simulink model "WOTC_simulation"  (R2024b)
settings: Solver=ode4  StartTime=0.0  StopTime=4700  FixedStep=0.01  RelTol=1e-3
InitFcn:
  | % Clear all variables from the workspace to ensure a clean start
  | clearvars;
  | 
  | % Run the setup script to load fresh parameters
  | run('models/osvData.m');
  | 
  | % Print a message to the command window to confirm
  | disp('Workspace cleared and initial variables loaded.');
StopFcn:
  | % Folder name
  | saveFolder = 'output data/';
  | timestamp = string(datetime('now', 'Format', 'yyyyMMdd_HHmmss'));
  | 
  | %make folder for simulation run data
  | mkdir(saveFolder + timestamp);
  | 
  | filePath = saveFolder + timestamp + "/" + timestamp + ".mat";
  | 
  | % 3. SAVE the file to the specified location
  | save(filePath, 'out');
  | 
  | disp(['Simulation data saved to: ' filePath]);
undefined symbols (not defined in the file or in its folder): osvData, vessel
libraries: wopc_lib x23, mssSimulink x6, simulink_extras x3, dspsigops x1, SignalEditorBlockLib x1
settings Model: PauseTimes=0  PacingRate=0.010000  Creator=lenna  LastModifiedBy=lenna
settings ModelReferenceCC: EnableRefExpFcnMdlSchedulingChecks=on

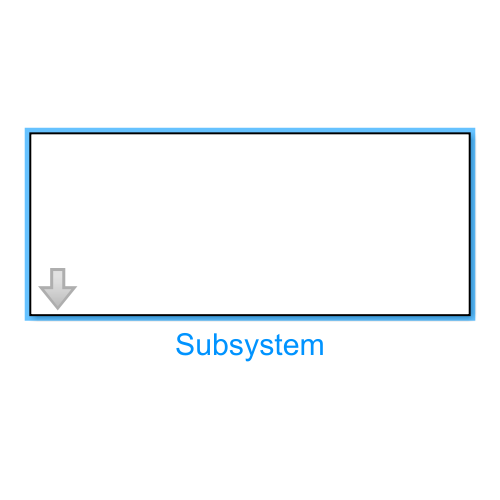
[thumbnail: Simulink's stored preview of the top-level diagram]
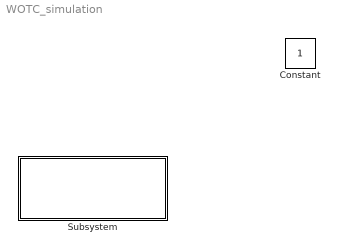
== system WOTC_simulation ==
  Subsystem : Subsystem  LoadFcn=osvData;  mask{eta0=[0 0 0]}
      mask prompts: eta0 "Initial position eta0"
  Constant : Constant  IOType=siggen

== system WOTC_simulation/Subsystem ==
  Controller : Subsystem
  Guidance : Subsystem
  Model : Subsystem
  wires:
  Model/1(eta) -> Controller/4(eta)  "eta"
  Model/2(nu) -> Controller/5(nu)  "nu"
  Guidance/1(etad) -> Controller/1(etad)  "etad"
  Guidance/2(etad_dot) -> Controller/2(etad_dot)  "etad_dot"
  Guidance/3(etad_ddot) -> Controller/3(etad_ddot)  "etad_ddot"
  Controller/1(tau) -> Model/1(tau)  "tau"

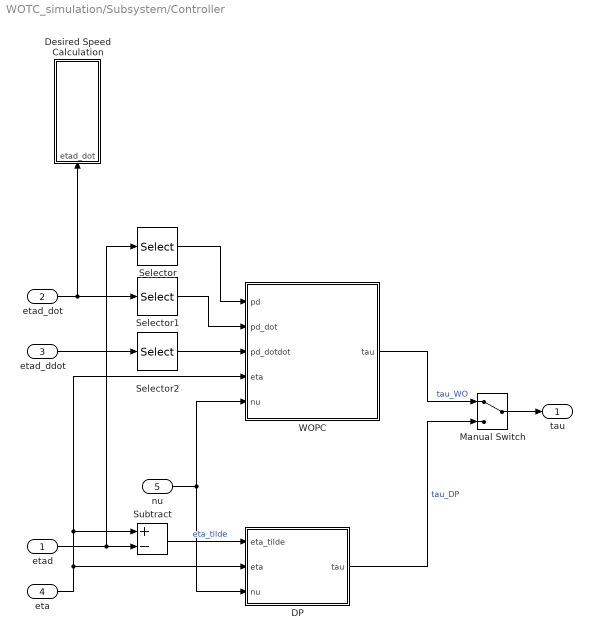
== system WOTC_simulation/Subsystem/Controller ==
  etad : Inport
  etad_dot : Inport  Port=2
  etad_ddot : Inport  Port=3
  eta : Inport  Port=4
  nu : Inport  Port=5
  DP : Subsystem
  Desired Speed Calculation : Subsystem
  Manual Switch : ManualSwitch
  Selector : Selector  InputPortWidth=3  IndexOptions=Index vector (dialog)  Indices=[1 2]  OutputSizes=1
  Selector1 : Selector  InputPortWidth=3  IndexOptions=Index vector (dialog)  Indices=[1 2]  OutputSizes=1
  Selector2 : Selector  InputPortWidth=3  IndexOptions=Index vector (dialog)  Indices=[1 2]  OutputSizes=1
  Subtract : Sum  Inputs=+-
  WOPC : Subsystem  mask{kp_1=1, kp_3=1, kd_1=1, kd_2=1, kd_3=1, lambda_1=1, lambda_3=1, rho_d=1000, k0=0.1, mu=100}
      mask prompts: kp_1 "kp(1)"; kp_3 "kp(3)"; kd_1 "Kd 1"; kd_2 "Kd 2"; kd_3 "Kd 3"; rho_d "rho_d. Circle radius"; k0 "k0 > 0. Gain deviation from desired location pd"; mu "mu. Gain change of env. force in surge"
      mask DialogControl Kp Prompt: Kp [3x3 diag kp1,kp3]
      mask DialogControl Kd Prompt: Kd [3x3 diag kd1,kd2,kd3]
      mask DialogControl Lambda Prompt: Lambda [3x3 diag lambda1,lambda3]
      mask DialogControl rho_k0 Prompt: rho_d, k0 and mu
  tau : Outport
  wires:
  etad_dot/1 -> Desired Speed Calculation/1(etad_dot), Selector1/1
  etad_ddot/1 -> Selector2/1
  etad/1 -> Selector/1, Subtract/2
  nu/1 -> DP/3(nu), WOPC/5(nu)
  Selector1/1 -> WOPC/2(pd_dot)
  eta/1 -> WOPC/4(eta), Subtract/1, DP/2(eta)
  Selector/1 -> WOPC/1(pd)
  Selector2/1 -> WOPC/3(pd_dotdot)
  Subtract/1 -> DP/1(eta_tilde)  "eta_tilde"
  DP/1(tau) -> Manual Switch/2  "tau_DP"
  WOPC/1(tau) -> Manual Switch/1  "tau_WO"
  Manual Switch/1 -> tau/1

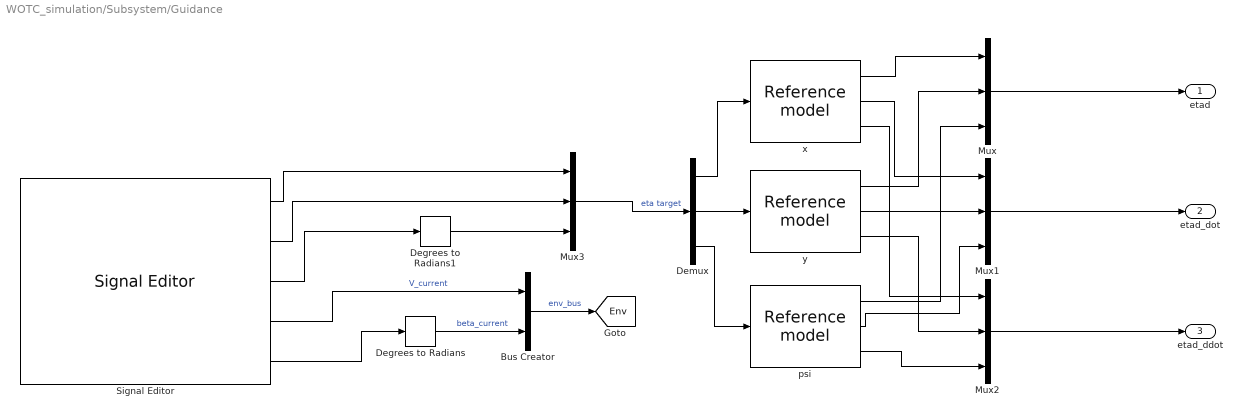
== system WOTC_simulation/Subsystem/Guidance ==
  Bus Creator : BusCreator  Inputs=2
  Degrees to Radians : simulink_extras/Transformations/Degrees to Radians
  Degrees to Radians1 : simulink_extras/Transformations/Degrees to Radians
  Demux : Demux  Outputs=3
  Mux{,1..3} (4 alike) : Mux  Inputs=3
  Signal Editor : SignalEditorBlockLib/Signal Editor  FileName=pipelineInspection_U1p5_Vc0p0_deg270.mat  ActiveScenario=pipelineInspection  ActiveSignal=eta_x  IsBus=off  OutputBusObjectStr=Bus: BusObject  SampleTime=0  ZeroCross=off  OutputAfterFinalValue=Holding final value  Unit=inherit  PreserveSignalName=on  ApplySigPropsToAllScenarios=on  ApplySigPropsToAllSignals=on
  psi : mssSimulink/Guidance/Reference model  v_max=0.035  zeta_d=1  w_d=0.1
      settings: SourceProductName=mss Toolbox
  x : mssSimulink/Guidance/Reference model  v_max=2.5  zeta_d=1.0  w_d=0.1
      settings: SourceProductName=mss Toolbox
  y : mssSimulink/Guidance/Reference model  v_max=2.5  zeta_d=1.0  w_d=0.1
      settings: SourceProductName=mss Toolbox
  etad : Outport
  etad_dot : Outport  Port=2
  etad_ddot : Outport  Port=3
  tag scope: Env=global
  wires:
  x/3 -> Mux2/1
  x/1 -> Mux/1
  Demux/1 -> x/1
  Demux/2 -> y/1
  Demux/3 -> psi/1
  y/1 -> Mux/2
  x/2 -> Mux1/1
  y/2 -> Mux1/2
  y/3 -> Mux2/2
  psi/1 -> Mux/3
  psi/2 -> Mux1/3
  psi/3 -> Mux2/3
  Mux3/1 -> Demux/1  "eta target"
  Signal Editor/1 -> Mux3/1
  Signal Editor/2 -> Mux3/2
  Degrees to Radians1/1 -> Mux3/3
  Signal Editor/3 -> Degrees to Radians1/1
  Signal Editor/4 -> Bus Creator/1  "V_current"
  Signal Editor/5 -> Degrees to Radians/1
  Bus Creator/1 -> [Env]  "env_bus"
  Degrees to Radians/1 -> Bus Creator/2  "beta_current"
  Mux/1 -> etad/1
  Mux1/1 -> etad_dot/1
  Mux2/1 -> etad_ddot/1

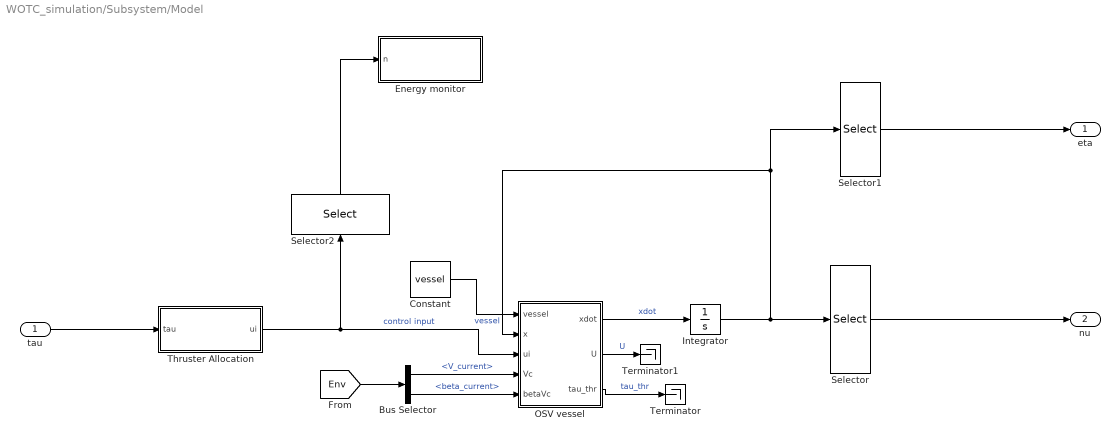
== system WOTC_simulation/Subsystem/Model ==
  tau : Inport
  Bus Selector : BusSelector  OutputSignals=V_current,beta_current
  Constant : Constant  Value=vessel  OutDataTypeStr=Bus: slBus1
  Energy monitor : Subsystem
  Integrator : Integrator  InitialCondition=[0 0 0 0 0 0 eta0(1) eta0(2) 0 0 0 eta0(3)]'
  OSV vessel : MATLAB Function  TreatAsAtomicUnit=on
  Selector : Selector  InputPortWidth=12  IndexOptions=Index vector (dialog)  Indices=[1 2 6]  OutputSizes=1
  Selector1 : Selector  InputPortWidth=12  IndexOptions=Index vector (dialog)  Indices=[7 8 12]  OutputSizes=1
  Selector2 : Selector  InputPortWidth=6  IndexOptions=Index vector (dialog)  Indices=[1 2 3 4]  OutputSizes=1
  Terminator : Terminator
  Terminator1 : Terminator
  Thruster Allocation : Subsystem
  eta : Outport
  nu : Outport  Port=2
  wires:
  Integrator/1 -> Selector/1, OSV vessel/2(x), Selector1/1
  Thruster Allocation/1(ui) -> Selector2/1, OSV vessel/3(ui)  "control input"
  Selector1/1 -> eta/1
  OSV vessel/1(xdot) -> Integrator/1  "xdot"
  Selector/1 -> nu/1
  tau/1 -> Thruster Allocation/1(tau)
  Constant/1 -> OSV vessel/1(vessel)  "vessel"
  [Env] -> Bus Selector/1
  Bus Selector/2 -> OSV vessel/5(betaVc)  "<beta_current>"
  Bus Selector/1 -> OSV vessel/4(Vc)  "<V_current>"
  OSV vessel/3(tau_thr) -> Terminator/1  "tau_thr"
  Selector2/1 -> Energy monitor/1(n)
  OSV vessel/2(U) -> Terminator1/1  "U"

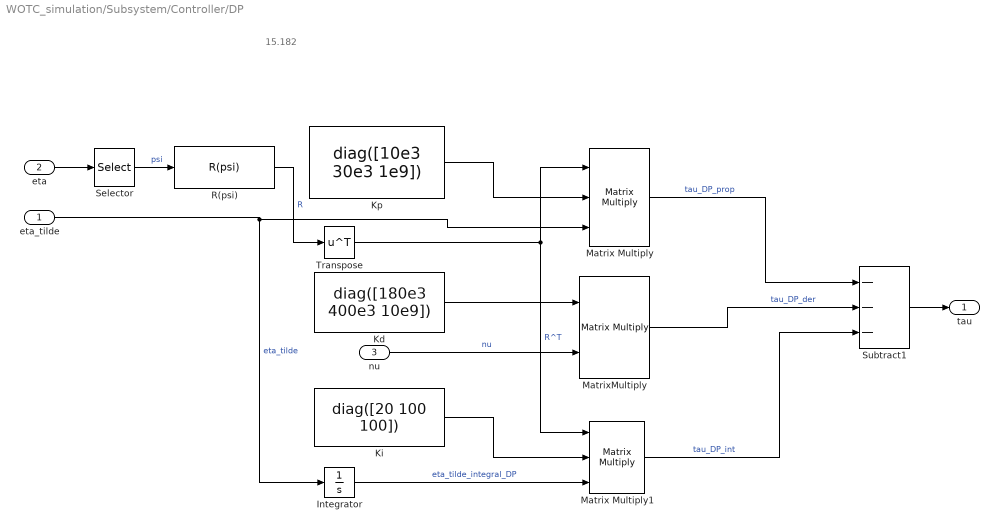
== system WOTC_simulation/Subsystem/Controller/DP ==
  note: 15.182
  eta_tilde : Inport
  eta : Inport  Port=2
  nu : Inport  Port=3
  Integrator : Integrator  InitialCondition=[0 0 0]'
  Kd : Constant  Value=diag([180e3 400e3 10e9])
  Ki : Constant  Value=diag([20 100 100])
  Kp : Constant  Value=diag([10e3 30e3 1e9])
  Matrix Multiply : Product  Inputs=3  Multiplication=Matrix(*)
  Matrix Multiply1 : Product  Inputs=3  Multiplication=Matrix(*)
  MatrixMultiply : Product  Multiplication=Matrix(*)
  R(psi) : wopc_lib/R(psi)  SystemSampleTime=-1  VariantActivationTime=update diagram  AllowFlexibleInterface=on  Latency=0  AutoFrameSizeCalculation=off
  Selector : Selector  InputPortWidth=3  IndexOptions=Index vector (dialog)  Indices=[3]  OutputSizes=1
  Subtract1 : Sum  Inputs=---
  Transpose : Math  Operator=transpose
  tau : Outport
  wires:
  eta/1 -> Selector/1
  Transpose/1 -> Matrix Multiply1/1, Matrix Multiply/1  "R^T"
  Selector/1 -> R(psi)/1  "psi"
  Kp/1 -> Matrix Multiply/2
  R(psi)/1 -> Transpose/1  "R"
  eta_tilde/1 -> Integrator/1, Matrix Multiply/3  "eta_tilde"
  Kd/1 -> MatrixMultiply/1
  nu/1 -> MatrixMultiply/2  "nu"
  Ki/1 -> Matrix Multiply1/2
  Integrator/1 -> Matrix Multiply1/3  "eta_tilde_integral_DP"
  Matrix Multiply/1 -> Subtract1/1  "tau_DP_prop"
  MatrixMultiply/1 -> Subtract1/2  "tau_DP_der"
  Matrix Multiply1/1 -> Subtract1/3  "tau_DP_int"
  Subtract1/1 -> tau/1

== system WOTC_simulation/Subsystem/Controller/Desired Speed Calculation ==
  etad_dot : Inport
  Add : Sum
  Demux : Demux  Outputs=3
  Square : Math  Operator=square
  Square Root : Sqrt
  Terminator : Terminator
  Terminator1 : Terminator
  wires:
  etad_dot/1 -> Square/1
  Demux/1 -> Add/1
  Square/1 -> Demux/1
  Demux/2 -> Add/2
  Demux/3 -> Terminator/1
  Add/1 -> Square Root/1
  Square Root/1 -> Terminator1/1  "Ud"

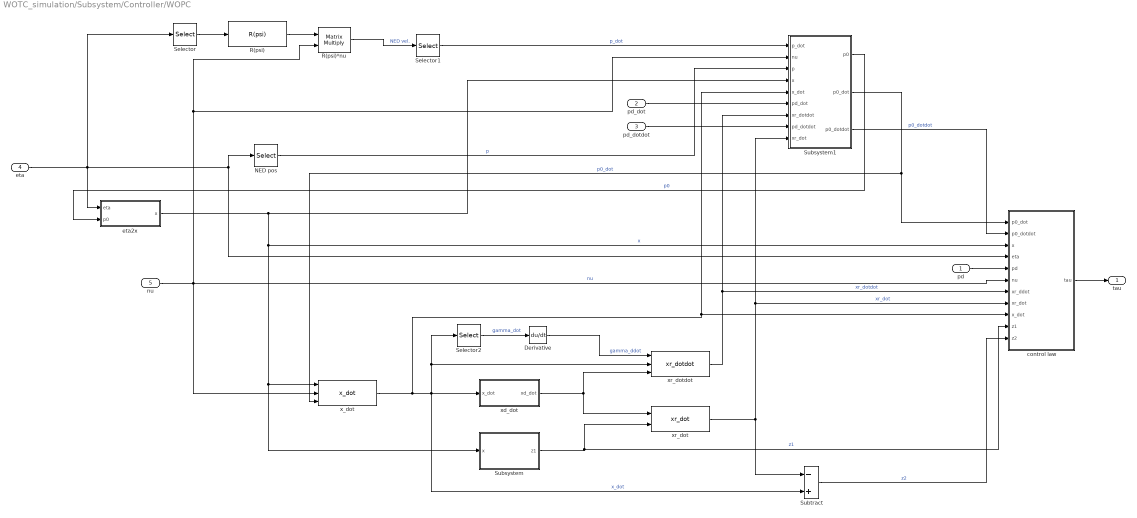
== system WOTC_simulation/Subsystem/Controller/WOPC ==
  pd : Inport
  pd_dot : Inport  Port=2
  pd_dotdot : Inport  Port=3
  eta : Inport  Port=4
  nu : Inport  Port=5  PortDimensions=3
  Derivative : Derivative
  NED pos : Selector  InputPortWidth=3  IndexOptions=Index vector (dialog)  Indices=[1 2]  OutputSizes=1
  R(psi) : wopc_lib/R(psi)  SystemSampleTime=-1  VariantActivationTime=update diagram  AllowFlexibleInterface=on  Latency=0  AutoFrameSizeCalculation=off
  R(psi)*nu : Product  Multiplication=Matrix(*)
  Selector : Selector  InputPortWidth=3  IndexOptions=Index vector (dialog)  Indices=3  OutputSizes=1
  Selector1 : Selector  InputPortWidth=3  IndexOptions=Index vector (dialog)  Indices=[1 2]  OutputSizes=1
  Selector2 : Selector  InputPortWidth=3  IndexOptions=Index vector (dialog)  Indices=2  OutputSizes=1
  Subsystem : Subsystem
  Subsystem1 : Subsystem
  Subtract : Sum  Inputs=-+
  control law : Subsystem
  eta2x : Subsystem
  x_dot : wopc_lib/x_dot  SystemSampleTime=-1  VariantActivationTime=update diagram  AllowFlexibleInterface=on  Latency=0  AutoFrameSizeCalculation=off
  xd_dot : Subsystem
  xr_dot : wopc_lib/xr_dot  SystemSampleTime=-1  VariantActivationTime=update diagram  AllowFlexibleInterface=on  Latency=0  AutoFrameSizeCalculation=off
  xr_dotdot : wopc_lib/xr_dotdot  SystemSampleTime=-1  VariantActivationTime=update diagram  AllowFlexibleInterface=on  Latency=0  AutoFrameSizeCalculation=off
  tau : Outport
  wires:
  eta/1 -> control law/4(eta), NED pos/1, Selector/1, eta2x/1(eta)
  pd/1 -> control law/5(pd)
  nu/1 -> x_dot/2, control law/6(nu), Subsystem1/2(nu), R(psi)*nu/2  "nu"
  eta2x/1(x) -> Subsystem1/4(x), Subsystem/1(x), x_dot/1, control law/3(x)  "x"
  Selector/1 -> R(psi)/1
  R(psi)/1 -> R(psi)*nu/1
  R(psi)*nu/1 -> Selector1/1  "NED vel."
  Subsystem/1(z1) -> control law/10(z1), xr_dot/2  "z1"
  xr_dot/1 -> Subsystem1/9(xr_dot), control law/8(xr_dot), Subtract/1  "xr_dot"
  x_dot/1 -> xd_dot/1(x_dot), Subtract/2, xr_dotdot/2, Selector2/1, Subsystem1/5(x_dot), control law/9(x_dot)  "x_dot"
  Subtract/1 -> control law/11(z2)  "z2"
  Subsystem1/1(p0) -> eta2x/2(p0)  "p0"
  Subsystem1/2(p0_dot) -> control law/1(p0_dot), x_dot/3  "p0_dot"
  Selector1/1 -> Subsystem1/1(p_dot)  "p_dot"
  NED pos/1 -> Subsystem1/3(p)  "p"
  pd_dot/1 -> Subsystem1/6(pd_dot)
  xr_dotdot/1 -> Subsystem1/7(xr_dotdot), control law/7(xr_ddot)  "xr_dotdot"
  pd_dotdot/1 -> Subsystem1/8(pd_dotdot)
  Subsystem1/3(p0_dotdot) -> control law/2(p0_dotdot)  "p0_dotdot"
  control law/1(tau) -> tau/1
  xd_dot/1(xd_dot) -> xr_dot/1, xr_dotdot/3
  Selector2/1 -> Derivative/1  "gamma_dot"
  Derivative/1 -> xr_dotdot/1  "gamma_ddot"

== system WOTC_simulation/Subsystem/Model/Energy monitor ==
  n : Inport
  Add : Sum  Inputs=++++
  Bus Selector : BusSelector  OutputSignals=K_thr
  Constant : Constant  Value=vessel  OutDataTypeStr=Bus: slBus1
  Demux : Demux
  Integrator : Integrator  InitialCondition=[0 0 0 0]'
  Matrix Multiply : Product  Multiplication=Matrix(*)
  Square : Math  Operator=square
  Terminator : Terminator
  wires:
  n/1 -> Square/1
  Constant/1 -> Bus Selector/1  "vessel"
  Bus Selector/1 -> Matrix Multiply/1  "<K_thr>"
  Matrix Multiply/1 -> Integrator/1  "thruster forces"
  Integrator/1 -> Demux/1  "tau_thr_individual"
  Demux/1 -> Add/1
  Demux/2 -> Add/2
  Demux/3 -> Add/3
  Demux/4 -> Add/4
  Add/1 -> Terminator/1  "tau_thr_sum"
  Square/1 -> Matrix Multiply/2

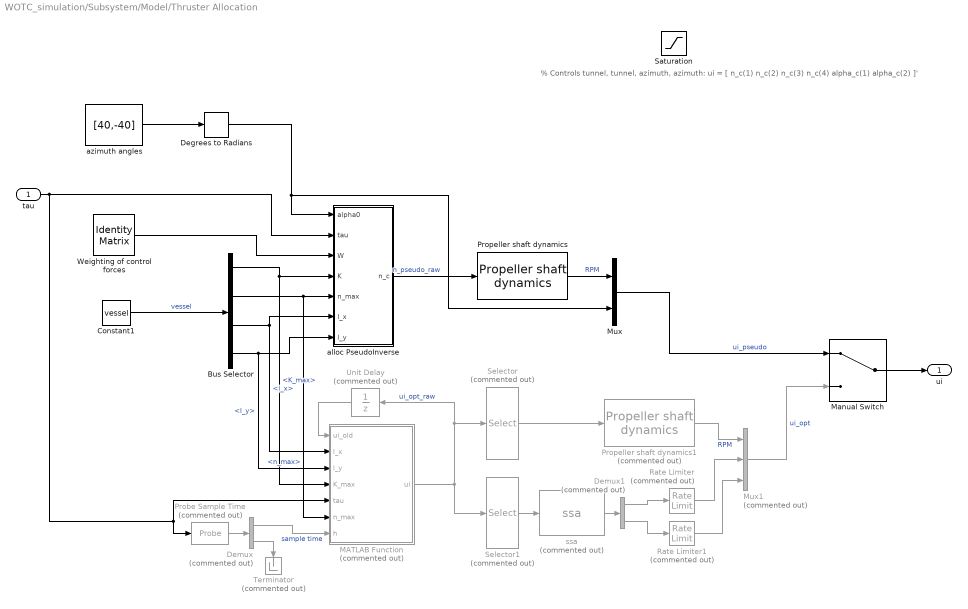
== system WOTC_simulation/Subsystem/Model/Thruster Allocation ==
  note: % Controls tunnel, tunnel, azimuth, azimuth:
      | ui = [ n_c(1) n_c(2) n_c(3) n_c(4) alpha_c(1) alpha_c(2) ]'
  tau : Inport
  Bus Selector : BusSelector  OutputSignals=K_max,n_max,l_x,l_y
  Constant1 : Constant  Value=vessel  OutDataTypeStr=Bus: slBus1
  Degrees to Radians : simulink_extras/Transformations/Degrees to Radians
  Demux : Demux  Commented=on  Outputs=2
  Demux1 : Demux  Commented=on  Outputs=2
  MATLAB Function : MATLAB Function  Commented=on  TreatAsAtomicUnit=on
  Manual Switch : ManualSwitch
  Mux : Mux  Inputs=2
  Mux1 : Mux  Commented=on  Inputs=3
  Probe Sample Time : Probe  Commented=on  ProbeWidth=off  ProbeComplexSignal=off
  Propeller shaft dynamics : mssSimulink/Modelling/Propulsion/Propeller shaft dynamics  rpm_max=150  rpm_rate=150/10  tc=1
      settings: SourceProductName=mss Toolbox
  Propeller shaft dynamics1 : mssSimulink/Modelling/Propulsion/Propeller shaft dynamics  Commented=on  rpm_max=150  rpm_rate=150/15  tc=1
      settings: SourceProductName=mss Toolbox
  Rate Limiter : RateLimiter  Commented=on  RisingSlewLimit=0.2  FallingSlewLimit=-0.2  SampleTimeMode=inherited  InitialCondition=deg2rad(60)
  Rate Limiter1 : RateLimiter  Commented=on  RisingSlewLimit=0.2  FallingSlewLimit=-0.2  SampleTimeMode=inherited  InitialCondition=deg2rad(-60)
  Saturation : Saturate  UpperLimit=150  LowerLimit=-150
  Selector : Selector  Commented=on  InputPortWidth=6  IndexOptions=Index vector (dialog)  Indices=[1 2 3 4]  OutputSizes=1
  Selector1 : Selector  Commented=on  InputPortWidth=6  IndexOptions=Index vector (dialog)  Indices=[5 6]  OutputSizes=1
  Terminator : Terminator  Commented=on
  Unit Delay : UnitDelay  Commented=on  InitialCondition=[0 0 0 0 deg2rad(90) deg2rad(-90)]'  SampleTime=-1  HasFrameUpgradeWarning=on
  Weighting of control forces : IdentityMatrix  OutputDimensions=4
  alloc PseudoInverse : MATLAB Function  TreatAsAtomicUnit=on
  azimuth angles : Constant  Value=[40,-40]
  ssa : mssSimulink/Utilities/Math Operations/ssa  Commented=on  SystemSampleTime=-1  VariantActivationTime=update diagram  AllowFlexibleInterface=on  Latency=0  AutoFrameSizeCalculation=off
      settings: SourceProductName=mss Toolbox
  ui : Outport
  wires:
  azimuth angles/1 -> Degrees to Radians/1
  Bus Selector/3 -> MATLAB Function/2(l_x), alloc PseudoInverse/6(l_x)  "<l_x>"
  Bus Selector/4 -> MATLAB Function/3(l_y), alloc PseudoInverse/7(l_y)  "<l_y>"
  Bus Selector/2 -> MATLAB Function/6(n_max), alloc PseudoInverse/5(n_max)  "<n_max>"
  Bus Selector/1 -> MATLAB Function/4(K_max), alloc PseudoInverse/4(K)  "<K_max>"
  tau/1 -> MATLAB Function/5(tau), Probe Sample Time/1, alloc PseudoInverse/2(tau)
  Constant1/1 -> Bus Selector/1  "vessel"
  Degrees to Radians/1 -> alloc PseudoInverse/1(alpha0), Mux/2
  Weighting of control forces/1 -> alloc PseudoInverse/3(W)
  Propeller shaft dynamics/1 -> Mux/1  "RPM"
  alloc PseudoInverse/1(n_c) -> Propeller shaft dynamics/1  "n_pseudo_raw"
  MATLAB Function/1(ui) -> Selector/1, Unit Delay/1, Selector1/1  "ui_opt_raw"
  Manual Switch/1 -> ui/1
  Mux/1 -> Manual Switch/1  "ui_pseudo"
  Unit Delay/1 -> MATLAB Function/1(ui_old)
  Probe Sample Time/1 -> Demux/1
  Demux/1 -> MATLAB Function/7(h)  "sample time"
  Demux/2 -> Terminator/1
  Selector/1 -> Propeller shaft dynamics1/1
  Rate Limiter/1 -> Mux1/2
  Propeller shaft dynamics1/1 -> Mux1/1  "RPM"
  Mux1/1 -> Manual Switch/2  "ui_opt"
  Selector1/1 -> ssa/1
  Demux1/1 -> Rate Limiter/1
  Demux1/2 -> Rate Limiter1/1
  Rate Limiter1/1 -> Mux1/3
  ssa/1 -> Demux1/1

== system WOTC_simulation/Subsystem/Controller/WOPC/Subsystem ==
  x : Inport
  Subtract : Sum  Inputs=+-
  pd2xd1 : Subsystem  AncestorBlock=wopc_lib/pd2xd
  z1 : Outport
  wires:
  pd2xd1/1(xd) -> Subtract/2
  Subtract/1 -> z1/1  "z1"
  x/1 -> pd2xd1/1(x), Subtract/1

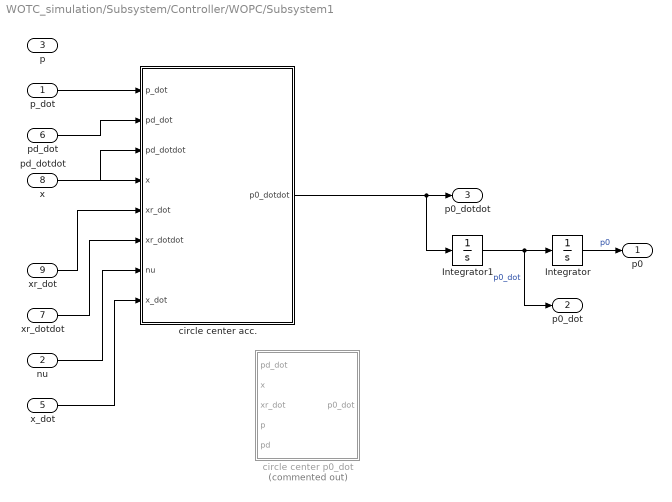
== system WOTC_simulation/Subsystem/Controller/WOPC/Subsystem1 ==
  p_dot : Inport
  nu : Inport  Port=2
  p : Inport  Port=3
  x : Inport  Port=4
  x_dot : Inport  Port=5
  pd_dot : Inport  Port=6
  xr_dotdot : Inport  Port=7
  pd_dotdot : Inport  Port=8
  xr_dot : Inport  Port=9
  Integrator : Integrator  InitialCondition=[eta0(1) + rho_d *cos(eta0(3));eta0(2)+rho_d*sin(eta0(3))]
  Integrator1 : Integrator  InitialCondition=[0;0]
  circle center acc. : Subsystem
  circle center p0_dot : Subsystem  Commented=on
  p0 : Outport
  p0_dot : Outport  Port=2
  p0_dotdot : Outport  Port=3
  wires:
  nu/1 -> circle center acc./7(nu)
  xr_dotdot/1 -> circle center acc./6(xr_dotdot)
  xr_dot/1 -> circle center acc./5(xr_dot)
  x/1 -> circle center acc./4(x)
  pd_dotdot/1 -> circle center acc./3(pd_dotdot)
  pd_dot/1 -> circle center acc./2(pd_dot)
  p_dot/1 -> circle center acc./1(p_dot)
  x_dot/1 -> circle center acc./8(x_dot)
  circle center acc./1(p0_dotdot) -> p0_dotdot/1, Integrator1/1
  Integrator1/1 -> p0_dot/1, Integrator/1  "p0_dot"
  Integrator/1 -> p0/1  "p0"

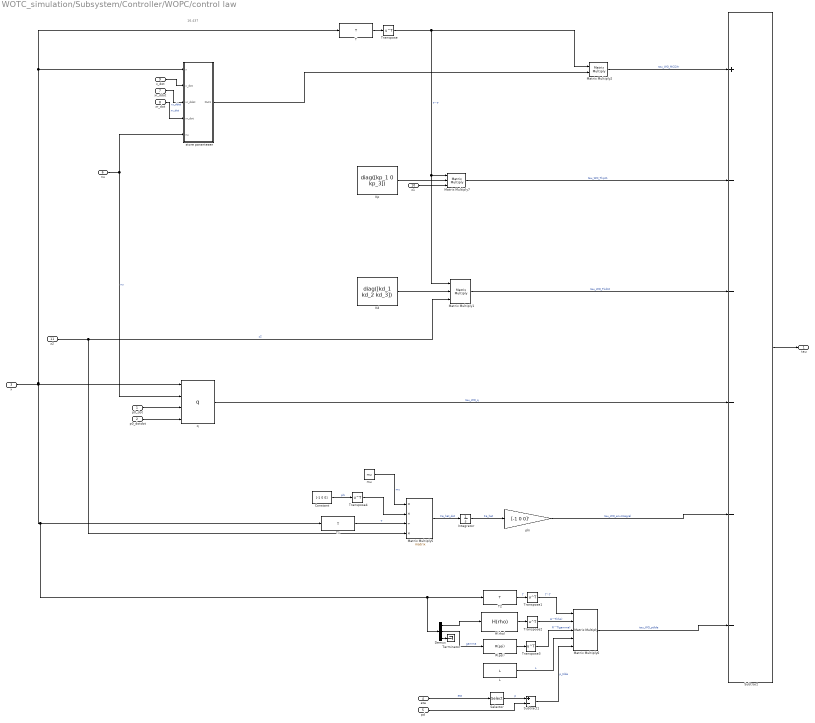
== system WOTC_simulation/Subsystem/Controller/WOPC/control law ==
  note: 16.437
  p0_dot : Inport
  p0_dotdot : Inport  Port=2
  x : Inport  Port=3
  eta : Inport  Port=4
  pd : Inport  Port=5
  nu : Inport  Port=6
  xr_ddot : Inport  Port=7
  xr_dot : Inport  Port=8
  x_dot : Inport  Port=9
  z1 : Inport  Port=10
  z2 : Inport  Port=11
  Constant : Constant  Value=[-1 0 0]
  Demux : Demux  Outputs=3
  H(rho) : wopc_lib/H(rho)  SystemSampleTime=-1  VariantActivationTime=update diagram  AllowFlexibleInterface=on  Latency=0  AutoFrameSizeCalculation=off
  Integrator : Integrator
  Kd : Constant  Value=diag([kd_1 kd_2 kd_3])
  Kp : Constant  Value=diag([kp_1 0 kp_3])
  L : wopc_lib/L  SystemSampleTime=-1  VariantActivationTime=update diagram  AllowFlexibleInterface=on  Latency=0  AutoFrameSizeCalculation=off
  Matrix Multiply1 : Product  Inputs=3  Multiplication=Matrix(*)
  Matrix Multiply2 : Product  Multiplication=Matrix(*)
  Matrix Multiply5 : Product  Inputs=**/*  Multiplication=Matrix(*)
  Matrix Multiply6 : Product  Inputs=5  Multiplication=Matrix(*)
  Matrix Multiply7 : Product  Inputs=3  Multiplication=Matrix(*)
  R(psi) : wopc_lib/R(psi)  SystemSampleTime=-1  VariantActivationTime=update diagram  AllowFlexibleInterface=on  Latency=0  AutoFrameSizeCalculation=off
  Selector : Selector  InputPortWidth=3  IndexOptions=Index vector (dialog)  Indices=[1 2]  OutputSizes=1
  Subtract : Sum  Inputs=+-----
  Subtract1 : Sum  Inputs=+-
  T : wopc_lib/T  SystemSampleTime=-1  VariantActivationTime=update diagram  AllowFlexibleInterface=on  Latency=0  AutoFrameSizeCalculation=off
  T1 : wopc_lib/T  SystemSampleTime=-1  VariantActivationTime=update diagram  AllowFlexibleInterface=on  Latency=0  AutoFrameSizeCalculation=off
  T2 : wopc_lib/T  SystemSampleTime=-1  VariantActivationTime=update diagram  AllowFlexibleInterface=on  Latency=0  AutoFrameSizeCalculation=off
  Terminator : Terminator
  Transpose{,1..4} (5 alike) : Math  Operator=transpose
  mu : Constant  Value=mu
  phi : Gain  Gain=[-1 0 0]'
  q : wopc_lib/q  SystemSampleTime=-1  VariantActivationTime=update diagram  AllowFlexibleInterface=on  Latency=0  AutoFrameSizeCalculation=off
      settings: AttributesFormatString=|
      | Bidrag fra flytting av sirkelsentrum p0
      | kompenserer for dette
  store parantesen : Subsystem
  tau : Outport
  wires:
  p0_dotdot/1 -> q/4
  p0_dot/1 -> q/3
  nu/1 -> store parantesen/5(nu), q/2  "nu"
  x/1 -> q/1, T1/1, Demux/1, T2/1, T/1, store parantesen/1(x)
  Subtract/1 -> tau/1
  q/1 -> Subtract/4  "tau_WO_q"
  T/1 -> Transpose/1
  Transpose/1 -> Matrix Multiply1/1, Matrix Multiply7/1, Matrix Multiply2/1  "T^T"
  Matrix Multiply2/1 -> Subtract/1  "tau_WO_MCDXr"
  mu/1 -> Matrix Multiply5/1  "mu"
  Constant/1 -> Transpose4/1  "phi"
  T1/1 -> Matrix Multiply5/3  "T"
  Matrix Multiply5/1 -> Integrator/1  "Fe_hat_dot"
  Integrator/1 -> phi/1  "Fe_hat"
  phi/1 -> Subtract/5  "tau_WO_envIntegral"
  eta/1 -> Selector/1  "eta"
  pd/1 -> Subtract1/2
  Selector/1 -> Subtract1/1  "p"
  Subtract1/1 -> Matrix Multiply6/5  "p_tilde"
  T2/1 -> Transpose1/1  "T"
  Transpose1/1 -> Matrix Multiply6/1  "T^T"
  H(rho)/1 -> Transpose2/1
  Transpose2/1 -> Matrix Multiply6/2  "H^T(rho)"
  R(psi)/1 -> Transpose3/1
  Transpose3/1 -> Matrix Multiply6/3  "R^T(gamma)"
  L/1 -> Matrix Multiply6/4  "L"
  Matrix Multiply6/1 -> Subtract/6  "tau_WO_ptilde"
  Demux/1 -> H(rho)/1
  Demux/2 -> R(psi)/1  "gamma"
  Demux/3 -> Terminator/1
  Transpose4/1 -> Matrix Multiply5/2
  x_dot/1 -> store parantesen/2(x_dot)
  xr_ddot/1 -> store parantesen/3(xr_ddot)  "xr_ddot"
  xr_dot/1 -> store parantesen/4(xr_dot)  "xr_dot"
  z2/1 -> Matrix Multiply1/3, Matrix Multiply5/4  "z2"
  store parantesen/1(Out1) -> Matrix Multiply2/2
  z1/1 -> Matrix Multiply7/3
  Kp/1 -> Matrix Multiply7/2
  Matrix Multiply7/1 -> Subtract/2  "tau_WO_Tkpz1"
  Matrix Multiply1/1 -> Subtract/3  "tau_WO_Tkdz2"
  Kd/1 -> Matrix Multiply1/2

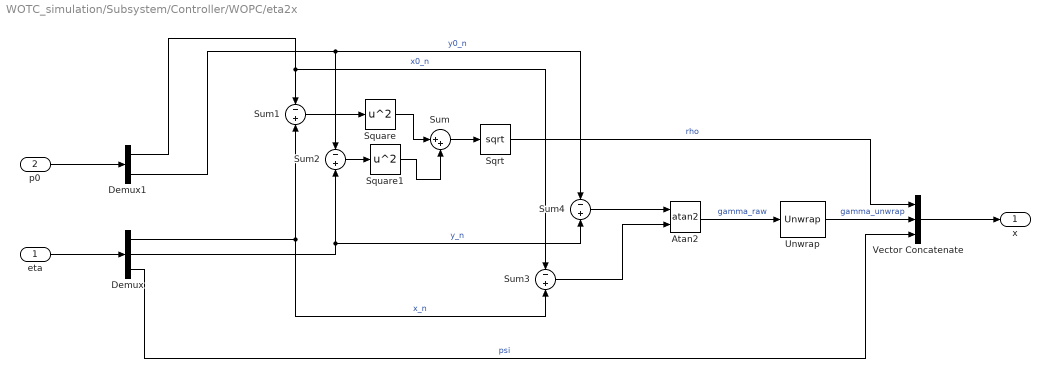
== system WOTC_simulation/Subsystem/Controller/WOPC/eta2x ==
  eta : Inport
  p0 : Inport  Port=2
  Atan2 : Trigonometry  Operator=atan2
  Demux : Demux  Outputs=3
  Demux1 : Demux  Outputs=2
  Sqrt : Sqrt
  Square : Math  Operator=square
  Square1 : Math  Operator=square
  Sum : Sum  Inputs=|++
  Sum{1..4} (4 alike) : Sum  Inputs=-+
  Unwrap : dspsigops/Unwrap  tol=pi  running=off
  Vector Concatenate : Concatenate  NumInputs=3
  x : Outport
  wires:
  Atan2/1 -> Unwrap/1  "gamma_raw"
  Sqrt/1 -> Vector Concatenate/1  "rho"
  Vector Concatenate/1 -> x/1
  eta/1 -> Demux/1
  Demux/3 -> Vector Concatenate/3  "psi"
  p0/1 -> Demux1/1
  Demux1/1 -> Sum3/1, Sum1/1  "x0_n"
  Demux/1 -> Sum3/2, Sum1/2  "x_n"
  Demux1/2 -> Sum4/1, Sum2/1  "y0_n"
  Demux/2 -> Sum4/2, Sum2/2  "y_n"
  Sum1/1 -> Square/1
  Sum2/1 -> Square1/1
  Square/1 -> Sum/1
  Square1/1 -> Sum/2
  Sum/1 -> Sqrt/1
  Sum4/1 -> Atan2/1
  Sum3/1 -> Atan2/2
  Unwrap/1 -> Vector Concatenate/2  "gamma_unwrap"

== system WOTC_simulation/Subsystem/Controller/WOPC/xd_dot ==
  x_dot : Inport
  Selector : Selector  InputPortWidth=3  IndexOptions=Index vector (dialog)  Indices=2  OutputSizes=1
  Vector Concatenate : Concatenate  NumInputs=3
  gamma_d : Constant  Value=0
  rho_d : Constant  Value=0
  xd_dot : Outport
  wires:
  x_dot/1 -> Selector/1
  rho_d/1 -> Vector Concatenate/1
  gamma_d/1 -> Vector Concatenate/2
  Vector Concatenate/1 -> xd_dot/1
  Selector/1 -> Vector Concatenate/3  "psi_d_dot = gamma_dot"

== system WOTC_simulation/Subsystem/Controller/WOPC/Subsystem/pd2xd1 ==
  note: x = [rho,gamma, psi] polar coord.
  x : Inport
  Add : Sum  Inputs=+-
  Constant : Constant  Value=pi
  Selector : Selector  InputPortWidth=3  IndexOptions=Index vector (dialog)  Indices=2  OutputSizes=1
  Vector Concatenate : Concatenate  NumInputs=3
  gamma_d : Constant  Value=0
  rho_d : Constant  Value=rho_d
  xd : Outport
  wires:
  Selector/1 -> Add/1  "gamma"
  x/1 -> Selector/1
  Add/1 -> Vector Concatenate/3  "psi_d"
  Constant/1 -> Add/2
  Vector Concatenate/1 -> xd/1
  rho_d/1 -> Vector Concatenate/1
  gamma_d/1 -> Vector Concatenate/2

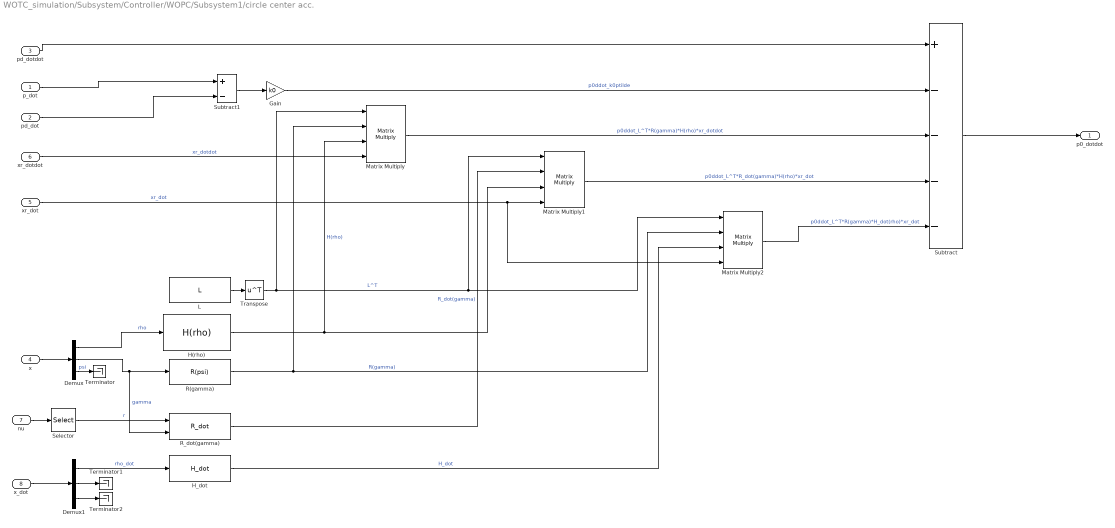
== system WOTC_simulation/Subsystem/Controller/WOPC/Subsystem1/circle center acc. ==
  p_dot : Inport
  pd_dot : Inport  Port=2
  pd_dotdot : Inport  Port=3
  x : Inport  Port=4
  xr_dot : Inport  Port=5
  xr_dotdot : Inport  Port=6
  nu : Inport  Port=7
  x_dot : Inport  Port=8
  Demux : Demux  Outputs=3
  Demux1 : Demux  Outputs=3
  Gain : Gain  Gain=k0
  H(rho) : wopc_lib/H(rho)  SystemSampleTime=-1  VariantActivationTime=update diagram  AllowFlexibleInterface=on  Latency=0  AutoFrameSizeCalculation=off
  H_dot : wopc_lib/H_dot  SystemSampleTime=-1  VariantActivationTime=update diagram  AllowFlexibleInterface=on  Latency=0  AutoFrameSizeCalculation=off
  L : wopc_lib/L  SystemSampleTime=-1  VariantActivationTime=update diagram  AllowFlexibleInterface=on  Latency=0  AutoFrameSizeCalculation=off
  Matrix Multiply : Product  Inputs=4  Multiplication=Matrix(*)
  Matrix Multiply1 : Product  Inputs=4  Multiplication=Matrix(*)
  Matrix Multiply2 : Product  Inputs=4  Multiplication=Matrix(*)
  R(gamma) : wopc_lib/R(psi)  SystemSampleTime=-1  VariantActivationTime=update diagram  AllowFlexibleInterface=on  Latency=0  AutoFrameSizeCalculation=off
  R_dot(gamma) : wopc_lib/R_dot  SystemSampleTime=-1  VariantActivationTime=update diagram  AllowFlexibleInterface=on  Latency=0  AutoFrameSizeCalculation=off
  Selector : Selector  InputPortWidth=3  IndexOptions=Index vector (dialog)  Indices=3  OutputSizes=1
  Subtract : Sum  Inputs=+----
  Subtract1 : Sum  Inputs=+-
  Terminator : Terminator
  Terminator1 : Terminator
  Terminator2 : Terminator
  Transpose : Math  Operator=transpose
  p0_dotdot : Outport
  wires:
  Subtract/1 -> p0_dotdot/1
  pd_dotdot/1 -> Subtract/1
  p_dot/1 -> Subtract1/1
  pd_dot/1 -> Subtract1/2
  Subtract1/1 -> Gain/1
  Gain/1 -> Subtract/2  "p0ddot_k0ptilde"
  x/1 -> Demux/1
  Demux/1 -> H(rho)/1  "rho"
  nu/1 -> Selector/1
  Selector/1 -> R_dot(gamma)/1  "r"
  R_dot(gamma)/1 -> Matrix Multiply1/2  "R_dot(gamma)"
  R(gamma)/1 -> Matrix Multiply/2, Matrix Multiply2/2  "R(gamma)"
  H(rho)/1 -> Matrix Multiply/3, Matrix Multiply1/3  "H(rho)"
  L/1 -> Transpose/1
  Transpose/1 -> Matrix Multiply/1, Matrix Multiply2/1, Matrix Multiply1/1  "L^T"
  Matrix Multiply/1 -> Subtract/3  "p0ddot_L^T*R(gamma)*H(rho)*xr_dotdot"
  xr_dotdot/1 -> Matrix Multiply/4  "xr_dotdot"
  Matrix Multiply1/1 -> Subtract/4  "p0ddot_L^T*R_dot(gamma)*H(rho)*xr_dot"
  xr_dot/1 -> Matrix Multiply2/4, Matrix Multiply1/4  "xr_dot"
  Demux/2 -> R_dot(gamma)/2, R(gamma)/1  "gamma"
  Demux/3 -> Terminator/1  "psi"
  H_dot/1 -> Matrix Multiply2/3  "H_dot"
  Matrix Multiply2/1 -> Subtract/5  "p0ddot_L^T*R(gamma)*H_dot(rho)*xr_dot"
  x_dot/1 -> Demux1/1
  Demux1/1 -> H_dot/1  "rho_dot"
  Demux1/2 -> Terminator1/1
  Demux1/3 -> Terminator2/1

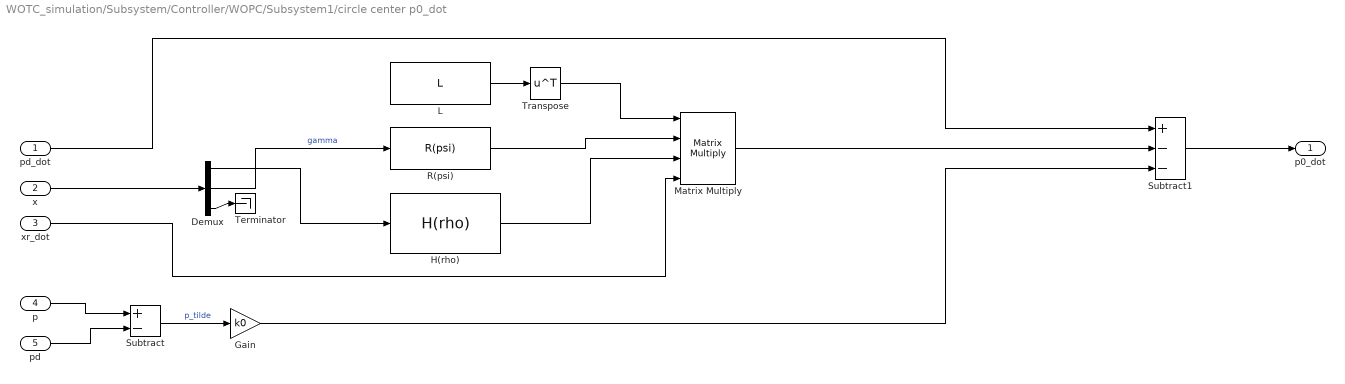
== system WOTC_simulation/Subsystem/Controller/WOPC/Subsystem1/circle center p0_dot ==
  pd_dot : Inport
  x : Inport  Port=2
  xr_dot : Inport  Port=3
  p : Inport  Port=4
  pd : Inport  Port=5
  Demux : Demux  Outputs=3
  Gain : Gain  Gain=k0
  H(rho) : wopc_lib/H(rho)  SystemSampleTime=-1  VariantActivationTime=update diagram  AllowFlexibleInterface=on  Latency=0  AutoFrameSizeCalculation=off
  L : wopc_lib/L  SystemSampleTime=-1  VariantActivationTime=update diagram  AllowFlexibleInterface=on  Latency=0  AutoFrameSizeCalculation=off
  Matrix Multiply : Product  Inputs=4  Multiplication=Matrix(*)
  R(psi) : wopc_lib/R(psi)  SystemSampleTime=-1  VariantActivationTime=update diagram  AllowFlexibleInterface=on  Latency=0  AutoFrameSizeCalculation=off
  Subtract : Sum  Inputs=+-
  Subtract1 : Sum  Inputs=+--
  Terminator : Terminator
  Transpose : Math  Operator=transpose
  p0_dot : Outport
  wires:
  p/1 -> Subtract/1
  pd/1 -> Subtract/2
  Subtract/1 -> Gain/1  "p_tilde"
  Subtract1/1 -> p0_dot/1
  Matrix Multiply/1 -> Subtract1/2
  L/1 -> Transpose/1
  Transpose/1 -> Matrix Multiply/1
  R(psi)/1 -> Matrix Multiply/2
  x/1 -> Demux/1
  Demux/1 -> H(rho)/1
  Demux/2 -> R(psi)/1  "gamma"
  Demux/3 -> Terminator/1
  xr_dot/1 -> Matrix Multiply/4
  H(rho)/1 -> Matrix Multiply/3
  Gain/1 -> Subtract1/3
  pd_dot/1 -> Subtract1/1

== system WOTC_simulation/Subsystem/Controller/WOPC/control law/store parantesen ==
  x : Inport
  x_dot : Inport  Port=2
  xr_ddot : Inport  Port=3
  xr_dot : Inport  Port=4
  nu : Inport  Port=5
  Add : Sum  Inputs=+++
  Cx : wopc_lib/Cx  SystemSampleTime=-1  VariantActivationTime=update diagram  AllowFlexibleInterface=on  Latency=0  AutoFrameSizeCalculation=off
  Dx : wopc_lib/Dx  SystemSampleTime=-1  VariantActivationTime=update diagram  AllowFlexibleInterface=on  Latency=0  AutoFrameSizeCalculation=off
  Matrix Multiply3 : Product  Multiplication=Matrix(*)
  Matrix Multiply4 : Product  Multiplication=Matrix(*)
  Matrix Multiply8 : Product  Multiplication=Matrix(*)
  Mx : wopc_lib/Mx  SystemSampleTime=-1  VariantActivationTime=update diagram  AllowFlexibleInterface=on  Latency=0  AutoFrameSizeCalculation=off
  Out1 : Outport
  wires:
  xr_ddot/1 -> Matrix Multiply3/2
  xr_dot/1 -> Matrix Multiply4/2, Matrix Multiply8/2
  Mx/1 -> Matrix Multiply3/1
  Matrix Multiply3/1 -> Add/1  "MxXr_ddot"
  nu/1 -> Cx/2, Dx/2
  Matrix Multiply8/1 -> Add/3  "DxXr_dot"
  Cx/1 -> Matrix Multiply4/1
  Dx/1 -> Matrix Multiply8/1  "Dx"
  Matrix Multiply4/1 -> Add/2  "CxXr_dot"
  x/1 -> Dx/1, Cx/1, Mx/1
  x_dot/1 -> Cx/3
  Add/1 -> Out1/1

== matlab function WOTC_simulation/Subsystem/Model/Thruster Allocation/MATLAB Function ==
  data: ui_old input; ui output; l_x input; l_y input; K_max input; tau input; n_max input; h input
function ui = optimal_alloc(ui_old,l_x,l_y, K_max,tau, n_max, h)

%test initial h step
if h == 0
    h = 0.0001;
end

% Get old azimuth angles and thruster commands from ui_old
u_old = ui_old(1:4);
alpha_old = ui_old(5:6);

% Dynamic optimization setup (if applicable)
%az_max = deg2rad(60);  % Max azimuth rotation angle (rad)

% Bounds for control variables:
%lb = [-az_max, -az_max, -1, -1, -1, -1, -inf, -inf, -inf];  % Lower bounds
%ub = [az_max, az_max, 1, 1, 1, 1, inf, inf, inf];           % Upper bounds
lb = [-pi, -pi, -1, -1, -1, -1, -inf, -inf, -inf];  % Lower bounds (no angle bound)
ub = [pi, pi, 1, 1, 1, 1, inf, inf, inf];           % Upper bounds (no angle bound)


% Constrained control allocation using dynamic optimization
[alpha_c, u_c, ~] = optimalAlloc(tau, lb, ub, alpha_old, ...
   u_old, l_x, l_y, K_max, h);


% Controls: ui = [ n_c(1) n_c(2) n_c(3) n_c(4) alpha_c(1) alpha_c(2) ]'
u_c = n_max.^2 .* u_c;  % Scale control efforts to actual propeller speeds
n_c = sign(u_c) .* sqrt(abs(u_c));  % Calculate each propeller's speed
ui = [n_c; alpha_c]; 

end

%% FUNCTIONS FOR DYNAMIC OPTIMIZATION
function [alpha_opt, u_opt, slack] = ...
    optimalAlloc(tau, lb, ub, alpha_old, u_old, l_x, l_y, K_thr, h)
% [alpha_opt, u_opt, slack] = ...
%    optimalAlloc(tau, lb, ub, alpha_old, u_old, l_x, l_y, K_thr, h)
% Constrained allocation is implemented by using sequential quadratic
% programming (SQP) to find the optimal (alpha, u) values when there
% are amplitude and rate saturations. The mathematical model is
%
% tau = T_thr(alpha) * K_thr * u
%   u = abs(n/n_max) * (n/n_max) - normalized squared propeller speed
%
% where the six controls are
%
% alpha = [alpha1, alpha2]'                        azimuth angles
% u = [bowAzimuth, starboardAzimuth, portAzimuth]  squared propeller speed
%
% Inputs:
%  tau: vector of generalized forces (surge, sway, yaw)
%  lb: vector of lower bounds
%  ub: vector of upper bounds
%  alpha_old: previous values of alpha
%  u_old: previous values of u
%  l_x: vector of x-coordinates, thruster lever arms
%  l_y: vector of y-coordinates, thruster lever arms
%  K_thr: diagonal matrix of maximum thrust
%  h: sampling time
%
% Outputs:
%  alpha_opt: optimal alpha values
%  u_opt: optimal u values, normalized
%  slack: norm of slack variables s = tau - T_thr(alpha) * K_thr * u
%
% Author:    Thor I. Fossen
% Date:      2024-03-25
% Revisions:

% Objective function
fun = @(x) objectiveFunction(x,alpha_old,u_old);

% Initial guess: x0 = [az1 az2 u1 u2 u3 u4 s1 s2 s3]
%x0 = [deg2rad(-28) deg2rad(28)  0 0 0 0  0 0 0];
x0 = [deg2rad(90) deg2rad(-90)  0 0 0 0  0 0 0];

% Use fmincon and sequential quadratic programming (SQP) to optimize
nonlcon = @(x) constraints(x, alpha_old, u_old, l_x, l_y, K_thr, tau, h);
options = optimoptions('fmincon','Display','off','Algorithm','sqp');
x_opt = fmincon(fun, x0, [], [], [], [], lb, ub, nonlcon, options);

% Extract results
alpha_opt = x_opt(1:2)';
u_opt = x_opt(3:6)';
slack = norm( x_opt(7:9) );

end

% Cost function
function cost = objectiveFunction(x,alpha_old,u_old)

alpha = x(1:2)';    % Azimuth angles
u = x(3:6)';        % Quadratic controls
s = x(7:9)';        % Slack variables: tau = T(alpha) * K_thr * u + s

w1 = 1;             % Weight for squared u
w2 = 100;           % Weight for squared slack variable s
w3 = 1;             % Weight for squared change in alpha
w4 = 0.1;           % Weight for squared change in u

cost = w1 * norm(u)^2 ...
    + w2 * norm(s)^2 ...
    + w3 * norm(alpha - alpha_old)^2 ...
    + w4 * norm(u - u_old)^2;

end

% Constraints
function [c, ceq] = constraints(x, alpha_old, u_old, l_x, l_y, K_thr,tau,h)

alpha = x(1:2)';     % Azimuth angles
u = x(3:6)';         % Quadratic controls
s = x(7:9)';         % Slack variables: tau = T(alpha) * K_thr * u + s

% Maximum azimuth angle and pitch rates
max_rate_alpha = 0.3;  % 0.3 rad/s = 17.2 deg/s
max_rate_u = 0.1;               

% Initialize c array for code generation
%c = zeros(12,1);
c = [];

% Separate positive and negative constraints to avoid abs
% c(1) = ( alpha(1) - alpha_old(1) ) / h - max_rate_alpha; % Positive constraint for alpha(1)
% c(2) = -( alpha(1) - alpha_old(1) ) / h - max_rate_alpha; % Negative constraint for alpha(1)
% 
% c(3) = ( alpha(2) - alpha_old(2) ) / h - max_rate_alpha; % Positive constraint for alpha(2)
% c(4) = -( alpha(2) - alpha_old(2) ) / h - max_rate_alpha; % Negative constraint for alpha(2)
% 
% c(5) = ( u(1) - u_old(1) ) / h - max_rate_u; % Positive constraint for u(1)
% c(6) = -( u(1) - u_old(1) ) / h - max_rate_u; % Negative constraint for u(1)
% 
% c(7) = ( u(2) - u_old(2) ) / h - max_rate_u; % Positive constraint for u(2)
% c(8) = -( u(2) - u_old(2) ) / h - max_rate_u; % Negative constraint for u(2)
% 
% c(9) = ( u(3) - u_old(3) ) / h - max_rate_u; % Positive constraint for u(3)
% c(10) = -( u(3) - u_old(3) ) / h - max_rate_u; % Negative constraint for u(3)
% 
% c(11) = ( u(4) - u_old(4) ) / h - max_rate_u; % Positive constraint for u(4)
% c(12) = -( u(4) - u_old(4) ) / h - max_rate_u; % Negative constraint for u(4)

% Equality constraint
T_alpha = thrConfig( {'T', 'T', alpha(1), alpha(2)}, l_x, l_y);

ceq = T_alpha * diag(K_thr) * u - tau + s;

end

== matlab function WOTC_simulation/Subsystem/Model/OSV vessel ==
  data: vessel input; x input; ui input; xdot output; U output; Vc input; betaVc input; tau_thr output
function [xdot, U, tau_thr] = fcn(vessel, x, ui, Vc, betaVc)

% Temp for testing. Dont pass tau directly from controller to model by
% setting skip to 0
tau = 0;
skip_alloc = 0;

[xdot,U,M, tau_thr] = osv_modified(vessel,x,ui,Vc,betaVc, tau, skip_alloc);
%[xdot, U, M, D] = supply(eta, tau);

== matlab function WOTC_simulation/Subsystem/Model/Thruster Allocation/alloc PseudoInverse ==
  data: alpha0 input; tau input; W input; K input; n_max input; n_c output; l_x input; l_y input
function n_c = fcn(alpha0,tau,W,K,n_max,l_x,l_y)
% Thrust allocation taken from simOSV in MSS toolbox
% tau 3DOF control forces
% alpha0 constant azimuth angles (rad)
% W diagonal weights of the control forces
% K vector of max propeller thrust (N)
% l_x, l_y thruster coordinates

K_max = diag(K); % Max thrust for each propeller (N)
                     
% Thruster configuration matrix
T_thr = thrConfig({'T', 'T', alpha0(1), alpha0(2)}, l_x, l_y);  

u_c = allocPseudoinverse(K_max,T_thr,W,tau);


u_c = n_max.^2 .* u_c;  % Scale control efforts to actual propeller speeds
n_c = sign(u_c) .* sqrt(abs(u_c));  % Calculate each propeller's speed
